simulink model "NotLin"  (Simulink 7.3)
settings: Solver=ode45  StartTime=0  StopTime=0.1
libraries: simulink x6
settings Model: Creator=Admin  LastModifiedBy=Администратор1
settings OptimizationCC: BooleanDataType=off  InitFltsAndDblsToZero=on
settings DebuggingCC: SaveWithParameterizedLinksMsg=none  SignalResolutionControl=TryResolveAllWithWarning  SolverPrmCheckMsg=none  MultiTaskDSMMsg=warning  MultiTaskCondExecSysMsg=none  StrictBusMsg=None
settings HardwareCC: TargetUnknown=on
settings RTWCC: IncludeERTFirstTime=on
settings GRTTargetCC: TargetFcnLib=ansi_tfl_tmw.mat

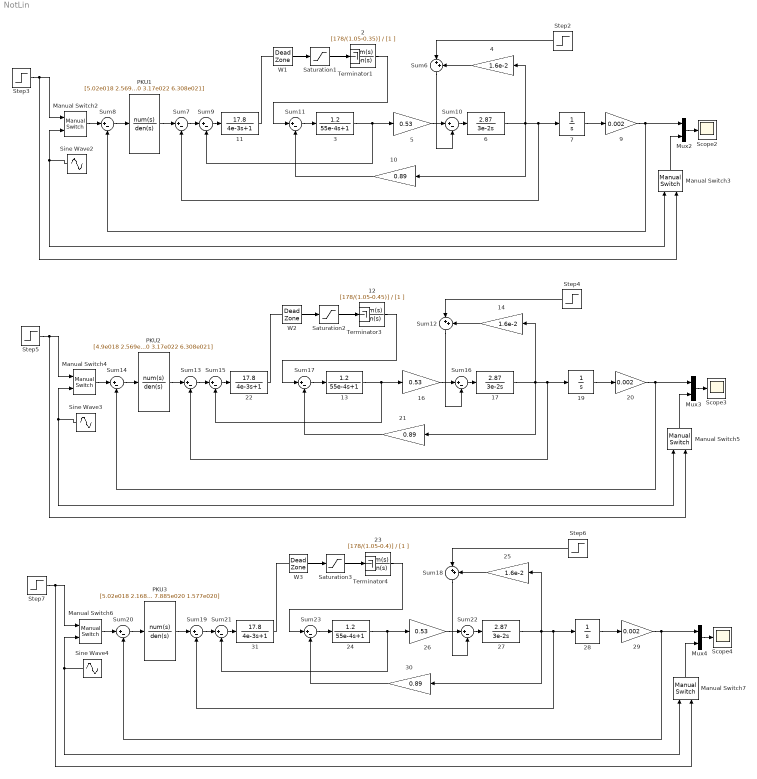
== system NotLin ==
  10 : Gain  Gain=0.89  ParameterDataType=sfix(16)  ParameterScaling=2^0  OutDataType=sfix(16)  OutScaling=2^0
  11 : TransferFcn  Numerator=[17.8]  Denominator=[4e-3 1]
  12 : TransferFcn  Numerator=[178/(1.05-0.45)]  Denominator=[1 ]
  13 : TransferFcn  Numerator=[1.2]  Denominator=[55e-4 1]
  14 : Gain  Gain=1.6e-2  ParameterDataType=sfix(16)  ParameterScaling=2^0  OutDataType=sfix(16)  OutScaling=2^0
  16 : Gain  Gain=0.53  ParameterDataType=sfix(16)  ParameterScaling=2^0  OutDataType=sfix(16)  OutScaling=2^0
  17 : TransferFcn  Numerator=[2.87]  Denominator=[3e-2 0]
  19 : TransferFcn  Numerator=[ 1 ]  Denominator=[1 0]
  2 : TransferFcn  Numerator=[178/(1.05-0.35)]  Denominator=[1 ]
  20 : Gain  Gain=0.002  ParameterDataType=sfix(16)  ParameterScaling=2^0  OutDataType=sfix(16)  OutScaling=2^0
  21 : Gain  Gain=0.89  ParameterDataType=sfix(16)  ParameterScaling=2^0  OutDataType=sfix(16)  OutScaling=2^0
  22 : TransferFcn  Numerator=[17.8]  Denominator=[4e-3 1]
  23 : TransferFcn  Numerator=[178/(1.05-0.4)]  Denominator=[1 ]
  24 : TransferFcn  Numerator=[1.2]  Denominator=[55e-4 1]
  25 : Gain  Gain=1.6e-2  ParameterDataType=sfix(16)  ParameterScaling=2^0  OutDataType=sfix(16)  OutScaling=2^0
  26 : Gain  Gain=0.53  ParameterDataType=sfix(16)  ParameterScaling=2^0  OutDataType=sfix(16)  OutScaling=2^0
  27 : TransferFcn  Numerator=[2.87]  Denominator=[3e-2 0]
  28 : TransferFcn  Numerator=[ 1 ]  Denominator=[1 0]
  29 : Gain  Gain=0.002  ParameterDataType=sfix(16)  ParameterScaling=2^0  OutDataType=sfix(16)  OutScaling=2^0
  3 : TransferFcn  Numerator=[1.2]  Denominator=[55e-4 1]
  30 : Gain  Gain=0.89  ParameterDataType=sfix(16)  ParameterScaling=2^0  OutDataType=sfix(16)  OutScaling=2^0
  31 : TransferFcn  Numerator=[17.8]  Denominator=[4e-3 1]
  4 : Gain  Gain=1.6e-2  ParameterDataType=sfix(16)  ParameterScaling=2^0  OutDataType=sfix(16)  OutScaling=2^0
  5 : Gain  Gain=0.53  ParameterDataType=sfix(16)  ParameterScaling=2^0  OutDataType=sfix(16)  OutScaling=2^0
  6 : TransferFcn  Numerator=[2.87]  Denominator=[3e-2 0]
  7 : TransferFcn  Numerator=[ 1 ]  Denominator=[1 0]
  9 : Gain  Gain=0.002  ParameterDataType=sfix(16)  ParameterScaling=2^0  OutDataType=sfix(16)  OutScaling=2^0
  Manual Switch2 : simulink/Signal Routing/Manual Switch  SystemSampleTime=-1  sw=1  action=0  varsize=off
  Manual Switch3 : simulink/Signal Routing/Manual Switch  SystemSampleTime=-1  sw=0  action=0  varsize=off
  Manual Switch4 : simulink/Signal Routing/Manual Switch  SystemSampleTime=-1  sw=1  action=0  varsize=off
  Manual Switch5 : simulink/Signal Routing/Manual Switch  SystemSampleTime=-1  sw=0  action=0  varsize=off
  Manual Switch6 : simulink/Signal Routing/Manual Switch  SystemSampleTime=-1  sw=1  action=0  varsize=off
  Manual Switch7 : simulink/Signal Routing/Manual Switch  SystemSampleTime=-1  sw=0  action=0  varsize=off
  Mux2 : Mux  Inputs=2
  Mux3 : Mux  Inputs=2
  Mux4 : Mux  Inputs=2
  PKU1 : TransferFcn  Numerator=[5.02e018 2.569e021 5.325e024 6.716e026 2.076e028 0]  Denominator=[0.09884 1.84e004 1.08e009 2.514e013 2.403e017 7.981e020 3.17e022 6.308e021]
  PKU2 : TransferFcn  Numerator=[4.9e018 2.569e021 5.325e024 6.716e026 2.076e028 0]  Denominator=[0.09884 1.84e004 1.08e009 2.514e013 2.403e017 7.981e020 3.17e022 6.308e021]
  PKU3 : TransferFcn  Numerator=[5.02e018 2.168e021 5.151e024 2.595e026 0]  Denominator=[0.09884 1.84e004 1.079e009 2.509e013 2.393e017 7.885e020 1.577e020]
  Saturation1 : Saturate  UpperLimit=178  LowerLimit=-178
  Saturation2 : Saturate  UpperLimit=178  LowerLimit=-178
  Saturation3 : Saturate  UpperLimit=178  LowerLimit=-178
  Scope2 : Scope
      settings: TickLabels=on  TimeRange=0.2  YMin=-1.1  YMax=1.1
  Scope3 : Scope
      settings: TickLabels=on  TimeRange=0.2  YMin=-1.1  YMax=1.1  SaveName=ScopeData2
  Scope4 : Scope
      settings: TickLabels=on  TimeRange=0.2  YMin=-1.1  YMax=1.1  SaveName=ScopeData3
  Sine Wave2 : Sin  Amplitude=1  Bias=0  Frequency=829.68  Phase=0  Samples=10  SampleTime=0  Offset=0
  Sine Wave3 : Sin  Amplitude=1  Bias=0  Frequency=896.4  Phase=0  Samples=10  SampleTime=0  Offset=0
  Sine Wave4 : Sin  Amplitude=1  Bias=0  Frequency=782.2  Phase=0  Samples=10  SampleTime=0  Offset=0
  Step2 : Step  Time=0  After=0.75  SampleTime=0
  Step3 : Step  Time=0  SampleTime=0
  Step4 : Step  Time=0  After=0.75  SampleTime=0
  Step5 : Step  Time=0  SampleTime=0
  Step6 : Step  Time=0  After=0.75  SampleTime=0
  Step7 : Step  Time=0  SampleTime=0
  Sum{7..11,13..17,19..23} (15 alike) : Sum  Inputs=|+-  OutDataType=sfix(16)  OutScaling=2^0
  Sum12 : Sum  Inputs=|++  OutDataType=sfix(16)  OutScaling=2^0
  Sum18 : Sum  Inputs=|++  OutDataType=sfix(16)  OutScaling=2^0
  Sum6 : Sum  Inputs=|++  OutDataType=sfix(16)  OutScaling=2^0
  Terminator1 : Terminator
  Terminator3 : Terminator
  Terminator4 : Terminator
  W1 : DeadZone  LowerValue=-0.35  UpperValue=+0.35  SaturateOnIntegerOverflow=on
  W2 : DeadZone  LowerValue=-0.45  UpperValue=+0.45  SaturateOnIntegerOverflow=on
  W3 : DeadZone  LowerValue=-0.40  UpperValue=+0.40  SaturateOnIntegerOverflow=on
  wires:
  Step3/1 -> Manual Switch2/1, Manual Switch3/2
  Sine Wave2/1 -> Manual Switch2/2, Manual Switch3/1
  Sum11/1 -> 3/1
  3/1 -> 5/1, Sum9/2
  6/1 -> 10/1, Sum7/2, 7/1, 4/1
  10/1 -> Sum11/2
  Mux2/1 -> Scope2/1
  9/1 -> Mux2/1, Sum8/2
  Manual Switch3/1 -> Mux2/2
  Manual Switch2/1 -> Sum8/1
  Sum7/1 -> Sum9/1
  Sum9/1 -> 11/1
  Sum8/1 -> PKU1/1
  5/1 -> Sum10/1
  Sum10/1 -> 6/1
  4/1 -> Sum6/2
  Step2/1 -> Sum6/1
  Sum6/1 -> Sum10/2
  7/1 -> 9/1
  W1/1 -> Saturation1/1
  PKU1/1 -> Sum7/1
  2/1 -> Terminator1/1, W1/1
  Saturation1/1 -> 2/1
  11/1 -> Sum11/1
  Step5/1 -> Manual Switch4/1, Manual Switch5/2
  Sine Wave3/1 -> Manual Switch4/2, Manual Switch5/1
  Sum17/1 -> 13/1
  13/1 -> 16/1, Sum15/2
  17/1 -> 21/1, Sum13/2, 19/1, 14/1
  21/1 -> Sum17/2
  Mux3/1 -> Scope3/1
  20/1 -> Mux3/1, Sum14/2
  Manual Switch5/1 -> Mux3/2
  Manual Switch4/1 -> Sum14/1
  Sum13/1 -> Sum15/1
  Sum15/1 -> 22/1
  Sum14/1 -> PKU2/1
  16/1 -> Sum16/1
  Sum16/1 -> 17/1
  14/1 -> Sum12/2
  Step4/1 -> Sum12/1
  Sum12/1 -> Sum16/2
  19/1 -> 20/1
  W2/1 -> Saturation2/1
  PKU2/1 -> Sum13/1
  12/1 -> Terminator3/1, W2/1
  Saturation2/1 -> 12/1
  22/1 -> Sum17/1
  Step7/1 -> Manual Switch6/1, Manual Switch7/2
  Sine Wave4/1 -> Manual Switch6/2, Manual Switch7/1
  Sum23/1 -> 24/1
  24/1 -> 26/1, Sum21/2
  27/1 -> 30/1, Sum19/2, 28/1, 25/1
  30/1 -> Sum23/2
  Mux4/1 -> Scope4/1
  29/1 -> Mux4/1, Sum20/2
  Manual Switch7/1 -> Mux4/2
  Manual Switch6/1 -> Sum20/1
  Sum19/1 -> Sum21/1
  Sum21/1 -> 31/1
  Sum20/1 -> PKU3/1
  26/1 -> Sum22/1
  Sum22/1 -> 27/1
  25/1 -> Sum18/2
  Step6/1 -> Sum18/1
  Sum18/1 -> Sum22/2
  28/1 -> 29/1
  W3/1 -> Saturation3/1
  PKU3/1 -> Sum19/1
  23/1 -> Terminator4/1, W3/1
  Saturation3/1 -> 23/1
  31/1 -> Sum23/1
